simulink model "TempoAcioProp"  (R2024a)
settings: Solver=FixedStepAuto  StartTime=0.0  StopTime=tf  FixedStep=step_modelo  RelTol=1e-3
settings Model: PacingRate=0.140000  Creator=rodri  LastModifiedBy=rodri
settings DataIOCC: SaveOutput=off  SaveTime=off
settings RTWCC: GPUComputeCapability=3.5

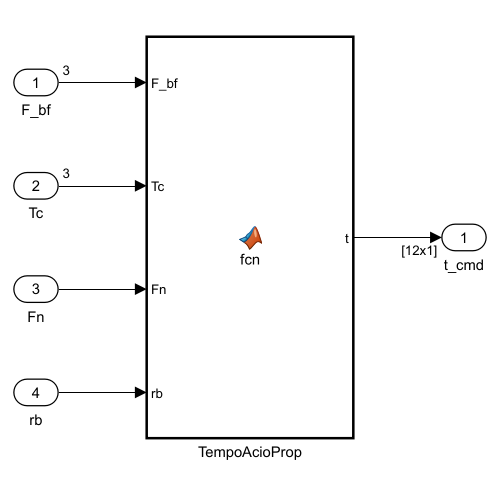
[thumbnail: Simulink's stored preview of the top-level diagram]
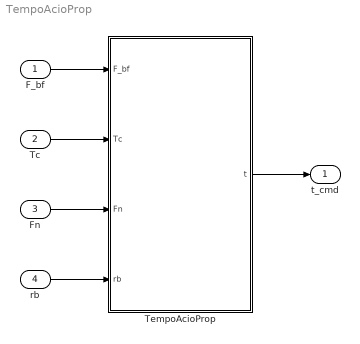
== system TempoAcioProp ==
  F_bf : Inport  OutDataTypeStr=double  PortDimensions=3
  Tc : Inport  Port=2  OutDataTypeStr=double  PortDimensions=3
  Fn : Inport  Port=3  OutDataTypeStr=double  PortDimensions=1
  rb : Inport  Port=4  OutDataTypeStr=double  PortDimensions=1
  TempoAcioProp : MATLAB Function  TreatAsAtomicUnit=on
  t_cmd : Outport  OutDataTypeStr=double  PortDimensions=[12 1]
  wires:
  F_bf/1 -> TempoAcioProp/1(F_bf)
  Tc/1 -> TempoAcioProp/2(Tc)
  Fn/1 -> TempoAcioProp/3(Fn)
  rb/1 -> TempoAcioProp/4(rb)
  TempoAcioProp/1(t) -> t_cmd/1

== matlab function TempoAcioProp/TempoAcioProp ==
  data: F_bf input; t output; Tc input; Fn input; rb input
function t = fcn(F_bf,Tc,Fn,rb)

Fx = F_bf(1);
Fy = F_bf(2);
Fz = F_bf(3);
Tx = Tc(1);
Ty = Tc(2);
Tz = Tc(3);

F = [Fx Fy Fz Tx Ty Tz]';

Tn = Fn*rb;

A = [Fn Fn 0 0 0 0 -Fn -Fn 0 0 0 0
    0 0 -Fn -Fn 0 0 0 0 Fn Fn 0 0
    0 0 0 0 -Fn -Fn 0 0 0 0 Fn Fn
    0 0 0 0 Tn -Tn 0 0 0 0 -Tn Tn
    -Tn Tn 0 0 0 0 Tn -Tn 0 0 0 0
    0 0 -Tn Tn 0 0 0 0 Tn -Tn 0 0];

c = [1 1 1 1 1 1 1 1 1 1 1 1];

[~,x] = nma_simplex(A,F,c,false);

t1 = x(1);
t2 = x(2);
t3 = x(3);
t4 = x(4);
t5 = x(5);
t6 = x(6);
t7 = x(7);
t8 = x(8);
t9 = x(9);
t10 = x(10);
t11 = x(11);
t12 = x(12);

if t1 < 0
    t7 = abs(t1);
    t1 = 0;
end

if t2 < 0
    t8 = abs(t2);
    t2 = 0;    
end

if t3 < 0
    t9 = abs(t3);
    t3 = 0;
end

if t4 < 0
    t10 = abs(t4);
    t4 = 0;
end

if t5 < 0
    t11 = abs(t5);
    t5 = 0;
end

if t6 < 0
    t12 = abs(t6);
    t6 = 0;
end

if t7 < 0
    t1 = abs(t7);
    t7 = 0;
end

if t8 < 0
    t2 = abs(t8);
    t8 = 0;
end

if t9 < 0
    t3 = abs(t9);
    t9 = 0;
end

if t10 < 0
    t4 = abs(t10);
    t10 = 0;
end

if t11 < 0
    t5 = abs(t11);
    t11 = 0;
end

if t12 < 0
    t6 = abs(t12);
    t12 = 0;
end

t = [t1;t2;t3;t4;t5;t6;t7;t8;t9;t10;t11;t12];

%Tese Willer
% A = [Fn Fn 0 0 0 0 -Fn -Fn 0 0 0 0
%     0 0 Fn Fn 0 0 0 0 -Fn -Fn 0 0
%     0 0 0 0 Fn Fn 0 0 0 0 -Fn -Fn
%     0 0 0 0 Tn -Tn 0 0 0 0 -Tn Tn
%     Tn -Tn 0 0 0 0 -Tn Tn 0 0 0 0
%     0 0 Tn -Tn 0 0 0 0 -Tn Tn 0 0];
